simulink model "master_pid_sys"  (R2015a)
settings: Solver=ode45  StartTime=0.0  StopTime=40  RelTol=1e-3
values from neighbouring files (symbols this model uses):
  A = [0 1; 0 -Bm/Mm]    [master_pid.m]
  B = [0; 1/Mm]    [master_pid.m]
  C = [1 0; 0 1]    [master_pid.m]
  D = [0; 0]    [master_pid.m]
  K = [5 5]    [master_pid.m]
settings Model: Creator=enrico-giordano  LastModifiedBy=enrico-giordano

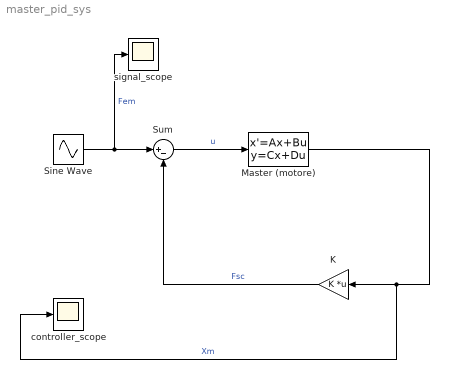
== system master_pid_sys ==
  K : Gain  Gain=K  Multiplication=Matrix(K*u)
  Master (motore) : StateSpace  A=A  B=B  C=C  D=D  X0=0
  Sine Wave : Sin  Amplitude=10  SampleTime=0
  Sum : Sum  Inputs=|+-
  controller_scope : Scope
      settings: TimeRange=10  YMin=-0.6000000000000001  YMax=0.2  SaveName=ScopeData3
  signal_scope : Scope
      settings: TimeRange=10  YMin=-10  YMax=10
  wires:
  Sum/1 -> Master (motore)/1  "u"
  Sine Wave/1 -> signal_scope/1, Sum/1  "Fem"
  Master (motore)/1 -> controller_scope/1, K/1  "Xm"
  K/1 -> Sum/2  "Fsc"
